simulink model "Test_Kinematics"  (R2024b)
settings: Solver=ode3  StartTime=0.0  StopTime=inf  FixedStep=.01  RelTol=1e-3  EnableMultiTasking=on
settings Model: Creator=GATEWAY
settings SolverCC: AlgebraicLoopSolver=TrustRegion
settings DataIOCC: LimitDataPoints=on  SaveFormat=Array  ReturnWorkspaceOutputs=off
settings OptimizationCC: LifeSpan=inf
settings DebuggingCC: UnderspecifiedInitializationDetection=Classic  MergeDetectMultiDrivingBlocksExec=none  SolverPrmCheckMsg=warning  UnconnectedInputMsg=warning  UnconnectedOutputMsg=warning  UnconnectedLineMsg=warning  StateNameClashWarn=warning  SFUnexpectedBacktrackingDiag=warning  SFNoUnconditionalDefaultTransitionDiag=warning  SFExecutionAtInitializationDiag=none  ArithmeticOperatorsInVariantConditions=warning
settings HardwareCC: ProdBitPerPointer=32  ProdBitPerSizeT=32  ProdBitPerPtrDiffT=32  ProdLargestAtomicFloat=None  ProdIntDivRoundTo=Undefined  ProdEndianess=Unspecified  ProdWordSize=32  ProdHWDeviceType=32-bit Generic
settings ModelReferenceCC: PropagateSignalLabelsOutOfModel=off
settings SFSimCC: SimUseLocalCustomCode=off  CustomCodeUndefinedFunction=UseInterfaceOnly
settings RTWCC: RTWUseLocalCustomCode=off  GPUComputeCapability=3.5
settings CodeAppCC: StateflowObjectComments=on
settings GRTTargetCC: TargetLangStandard=C89/C90 (ANSI)
settings ConfigComp: CovMetricSettings=dw  CovSaveCumulativeToWorkspaceVar=on  CovSaveSingleToWorkspaceVar=on  CovExternalEMLEnable=off

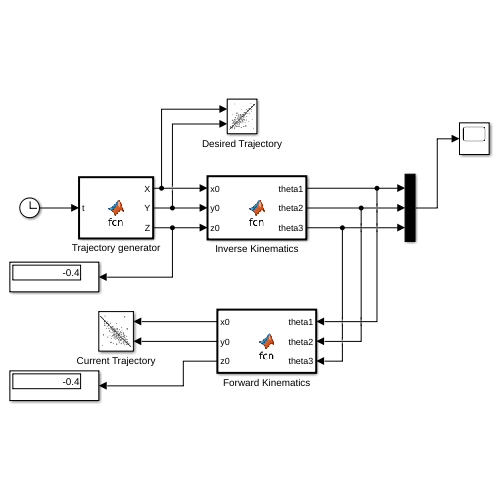
[thumbnail: Simulink's stored preview of the top-level diagram]
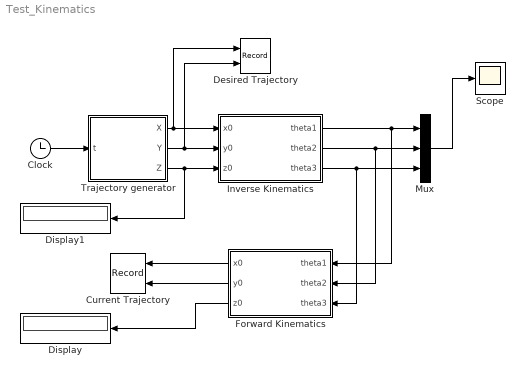
== system Test_Kinematics ==
  Clock : Clock
  Current Trajectory : Record  FileSettingsInternal="{\"entries\":[{\"content\":{\"excelSettings\":{\"content\":{},\"type\":\"Streamout.ExcelSettings\"}},\"type\":\"Streamout.FileSettingStorage\",\"uuid\":\"\"}],\"packageUris\":[\"http:\\/\\/schema.mathworks.com\\/mf0\\/streamout_blocks\\/R2020a\"],\"version\":\"1.0\"}"  Layout=[1 1]  SignalsInternal="{\"entries\":[{\"content\":{\"signals\":[{\"content\":{\"blockPath\":[],\"dimensions\":[1],\"domain\":\"\",\"lineColor\":\"#a2142f\",\"plots\":[ 1 ],\"port\":1,\"sid\":[\"\"],\"signalID\":1,\"signalName\":\"Forward Kinematics:1\"},\"type\":\"RecordBlkView.Signal\",\"uuid\":\"\"},{\"content\":{\"blockPath\":[],\"dimensions\":[1],\"domain\":\"\",\"lineColor\":\"#139fff\",\"plots\":[ 1 ],\"port\":2,\"sid\":[\"\"],\"signalID\":2,\"signalName\":\"Forward Kinematics:2\"},\"type\":\"RecordBlkView.Signal\",\"uuid\":\"\"}]},\"type\":\"RecordBlkView.InputSignals\",\"uuid\":\"\"}],\"packageUris\":[\"http:\\/\\/schema.mathworks.com\\/mf0\\/streamout_blocks\\/R2020a\"],\"version\":\"1.0\"}"  VisualizationBindings="{\"xyplotplugin\":{\"info\":[{\"series\":[{\"bindingParametersList\":[{\"parameter\":\"X-Axis\",\"signalID\":1,\"signalName\":\"Forward Kinematics:1\"},{\"parameter\":\"Y-Axis\",\"signalID\":2,\"signalName\":\"Forward Kinematics:2\"}],\"seriesID\":0}],\"subplotID\":1}]}}"  CompatibilityTag=XY  st=-1
  Desired Trajectory : Record  FileSettingsInternal="{\"entries\":[{\"content\":{\"excelSettings\":{\"content\":{},\"type\":\"Streamout.ExcelSettings\"}},\"type\":\"Streamout.FileSettingStorage\",\"uuid\":\"\"}],\"packageUris\":[\"http:\\/\\/schema.mathworks.com\\/mf0\\/streamout_blocks\\/R2020a\"],\"version\":\"1.0\"}"  Layout=[1 1]  SignalsInternal="{\"entries\":[{\"content\":{\"signals\":[{\"content\":{\"blockPath\":[],\"dimensions\":[1],\"domain\":\"\",\"lineColor\":\"#a2142f\",\"plots\":[ 1 ],\"port\":1,\"sid\":[\"\"],\"signalID\":1,\"signalName\":\"Trajectory generator:1\"},\"type\":\"RecordBlkView.Signal\",\"uuid\":\"\"},{\"content\":{\"blockPath\":[],\"dimensions\":[1],\"domain\":\"\",\"lineColor\":\"#139fff\",\"plots\":[ 1 ],\"port\":2,\"sid\":[\"\"],\"signalID\":2,\"signalName\":\"Trajectory generator:2\"},\"type\":\"RecordBlkView.Signal\",\"uuid\":\"\"}]},\"type\":\"RecordBlkView.InputSignals\",\"uuid\":\"\"}],\"packageUris\":[\"http:\\/\\/schema.mathworks.com\\/mf0\\/streamout_blocks\\/R2020a\"],\"version\":\"1.0\"}"  VisualizationBindings="{\"xyplotplugin\":{\"info\":[{\"series\":[{\"bindingParametersList\":[{\"parameter\":\"X-Axis\",\"signalID\":1,\"signalName\":\"Trajectory generator:1\"},{\"parameter\":\"Y-Axis\",\"signalID\":2,\"signalName\":\"Trajectory generator:2\"}],\"seriesID\":0}],\"subplotID\":1}]}}"  CompatibilityTag=XY  st=-1
  Display : Display
  Display1 : Display
  Forward Kinematics : MATLAB Function  TreatAsAtomicUnit=on
  Inverse Kinematics : MATLAB Function  TreatAsAtomicUnit=on
  Mux : Mux  Inputs=3
  Scope : Scope
  Trajectory generator : MATLAB Function  TreatAsAtomicUnit=on
  wires:
  Clock/1 -> Trajectory generator/1(t)
  Trajectory generator/1(X) -> Desired Trajectory/1, Inverse Kinematics/1(x0)
  Trajectory generator/2(Y) -> Desired Trajectory/2, Inverse Kinematics/2(y0)
  Trajectory generator/3(Z) -> Display1/1, Inverse Kinematics/3(z0)
  Mux/1 -> Scope/1
  Forward Kinematics/2(y0) -> Current Trajectory/2
  Inverse Kinematics/1(theta1) -> Forward Kinematics/1(theta1), Mux/1
  Forward Kinematics/1(x0) -> Current Trajectory/1
  Inverse Kinematics/3(theta3) -> Forward Kinematics/3(theta3), Mux/3
  Forward Kinematics/3(z0) -> Display/1
  Inverse Kinematics/2(theta2) -> Forward Kinematics/2(theta2), Mux/2

== matlab function Test_Kinematics/Trajectory generator ==
  data: t input; X output; Y output; Z output
function [X,Y,Z] = fcn(t)
% Circle plot as parametric curve
X = .1*cos(t);
Y = .1*sin(t);
Z = -.40;
end

== matlab function Test_Kinematics/Inverse Kinematics ==
  data: x0 input; theta1 output; y0 input; z0 input; theta2 output; theta3 output
function [theta1,theta2,theta3] = fcn(x0,y0,z0)
%Rotation of 120° en Z
x1= x0*cosd(120) + y0*sind(120);
y1=-x0*sind(120) + y0*cosd(120);
%Rotation of -120° en Z
x2= x0*cosd(120) - y0*sind(120);
y2= x0*sind(120) + y0*cosd(120);

%Compute theta 1
theta1=InverseKin(x0,y0,z0);
%Compute theta 2
theta2=InverseKin(x1,y1,z0);
%Compute theta 3
theta3=InverseKin(x2,y2,z0);

end

== matlab function Test_Kinematics/Forward Kinematics ==
  data: x0 output; theta1 input; y0 output; z0 output; theta2 input; theta3 input
function [x0,y0,z0] = fcn(theta1,theta2,theta3)
% Compute Forward Kinematics
[x,y,z]=ForwardKin(theta1,theta2,theta3);
x0=x;
y0=y;
z0=z;
end
